simulink model "raspberrypi_audioVisualizer"  (R2018b)
settings: Solver=ode3  StartTime=0.0  StopTime=10  RelTol=1e-3  EnableMultiTasking=on
libraries: dspmtrx3 x2, sensehatlib x1, embdlinuxlib x1, raspberrypilib x1, dspxfrm3 x1
settings Model: FPTRunName=Active  ExtModeTrigDuration=2  Creator=The MathWorks, Inc.  LastModifiedBy=The MathWorks, Inc.
settings SolverCC: PositivePriorityOrder=on
settings DataIOCC: LimitDataPoints=on  SaveFormat=Array
settings OptimizationCC: ExpressionDepthLimit=2147483647  LifeSpan=Inf  MaxStackSize=64
settings DebuggingCC: UnderspecifiedInitializationDetection=Classic  MergeDetectMultiDrivingBlocksExec=none  FcnCallInpInsideContextMsg=warning  AllowSymbolicDim=off  StateNameClashWarn=warning  SFUnexpectedBacktrackingDiag=warning  SFNoUnconditionalDefaultTransitionDiag=warning  SFExecutionAtInitializationDiag=none
settings HardwareCC: ProdBitPerPointer=32  ProdBitPerSizeT=32  ProdBitPerPtrDiffT=32  ProdLargestAtomicInteger=Long  ProdLargestAtomicFloat=Double  ProdWordSize=32  ProdHWDeviceType=ARM Compatible->ARM Cortex  UseEmbeddedCoderFeatures=off  UseSimulinkCoderFeatures=off
settings ModelReferenceCC: PropagateSignalLabelsOutOfModel=off
settings SFSimCC: SimUseLocalCustomCode=off
settings RTWCC: SystemTargetFile=ert.tlc  HardwareBoard=Raspberry Pi  TemplateMakefile=ert_default_tmf  GenerateReport=on  RTWVerbose=off  RTWUseLocalCustomCode=off  Toolchain=GNU GCC Raspberry Pi  BuildConfiguration=Faster Runs  LaunchReport=on
settings CodeAppCC: ForceParamTrailComments=on  OperatorAnnotations=on  StateflowObjectComments=on  MATLABSourceComments=on
settings ERTTargetCC: MultiwordLength=2048  ERTCustomFileBanners=off  SupportContinuousTime=on  SupportNonInlinedSFcns=on  RemoveResetFunc=off  SupportVariableSizeSignals=on  ModelStepFunctionPrototypeControlCompliant=off
settings ConfigComp: CovMetricSettings=dw  CovHtmlReporting=on  CovSaveCumulativeToWorkspaceVar=on  CovSaveSingleToWorkspaceVar=on  CovExternalEMLEnable=off  CovSFcnEnable=off

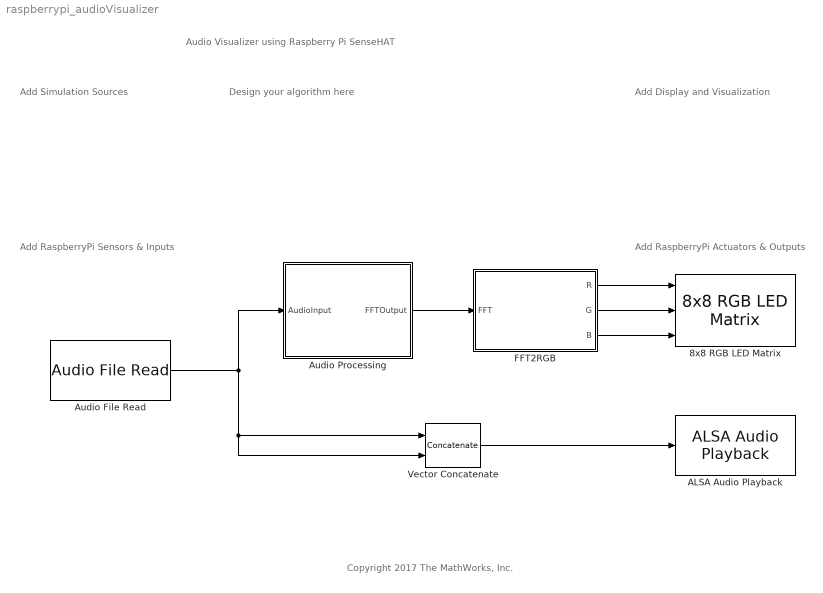
== system raspberrypi_audioVisualizer ==
  note: Copyright 2017 The MathWorks, Inc.
  note: Add Simulation Sources
  note: Add Display and Visualization
  note: Design your algorithm here
  note: Add RaspberryPi Actuators & Outputs
  note: Audio Visualizer using Raspberry Pi SenseHAT
  note: Add RaspberryPi Sensors & Inputs
  8x8 RGB LED Matrix : sensehatlib/8x8 RGB LED Matrix   Mode=Display Image  ImageSource=Separate color signals  OrientationSource=Block dialog  LEDOrientation=0  blockPlatform=Raspberry pi
      settings: SourceProductName=Simulink Support Package for Raspberry Pi Hardware  SourceProductBaseCode=RASPPI
  ALSA Audio Playback : embdlinuxlib/ALSA Audio Playback  deviceStr='hw:0,0'  sampleRateEnum=44100  queueDuration=0.5  blockPlatform=Raspberry Pi
      settings: SourceProductName=Simulink Support Package for Raspberry Pi Hardware  SourceProductBaseCode=RASPPI
  Audio File Read : raspberrypilib/Audio File Read  FileName=guitartune.wav  PlayCount=Inf  OutputEOFIndicator=off  SamplesPerFrame=8192
      settings: SourceProductName=Simulink Support Package for Raspberry Pi Hardware  SourceProductBaseCode=RASPPI
  Audio Processing : Subsystem
  FFT2RGB : MATLAB Function  TreatAsAtomicUnit=on
  Vector Concatenate : Concatenate  Mode=Multidimensional array  ConcatenateDimension=2
  wires:
  Audio File Read/1 -> Vector Concatenate/2, Vector Concatenate/1, Audio Processing/1(AudioInput)
  Vector Concatenate/1 -> ALSA Audio Playback/1
  FFT2RGB/1(R) -> 8x8 RGB LED Matrix/1
  FFT2RGB/2(G) -> 8x8 RGB LED Matrix/2
  FFT2RGB/3(B) -> 8x8 RGB LED Matrix/3
  Audio Processing/1(FFTOutput) -> FFT2RGB/1(FFT)

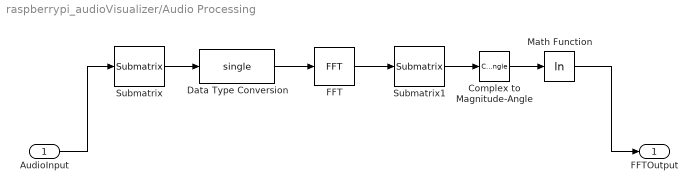
== system raspberrypi_audioVisualizer/Audio Processing ==
  AudioInput : Inport
  Complex to Magnitude-Angle : ComplexToMagnitudeAngle  Output=Magnitude
  Data Type Conversion : DataTypeConversion  OutDataTypeStr=single
  FFT : dspxfrm3/FFT  FFTImplementation=Auto  CompMethod=Table lookup  TableOpt=NEW  TableOptActive=Speed  BitRevOrder=off  Normalize=on  InheritFFTLength=on  FFTLength=64  WrapInput=on  roundingMode=Floor  overflowMode=off  firstCoeffDataTypeStr=Inherit: Same word length as input  firstCoeffLastDataTypeStr=Inherit: Same word length as input  outputMin=[]  outputMax=[]
  Math Function : Math  Operator=log  SaturateOnIntegerOverflow=on
  Submatrix : dspmtrx3/Submatrix  RowSpan=Range of rows  RowStartMode=First  RowStartIndex=1  RowEndMode=Last  RowEndIndex=1  ColSpan=One column  ColStartMode=First  ColStartIndex=1  ColEndMode=Last  ColEndIndex=1
  Submatrix1 : dspmtrx3/Submatrix  RowSpan=Range of rows  RowStartMode=Index  RowStartIndex=128  RowEndMode=Index  RowEndIndex=1151  ColSpan=Range of columns  ColStartMode=First  ColStartIndex=1  ColEndMode=Last  ColEndIndex=1
  FFTOutput : Outport
  wires:
  AudioInput/1 -> Submatrix/1
  Submatrix/1 -> Data Type Conversion/1
  Data Type Conversion/1 -> FFT/1
  FFT/1 -> Submatrix1/1
  Submatrix1/1 -> Complex to Magnitude-Angle/1
  Math Function/1 -> FFTOutput/1
  Complex to Magnitude-Angle/1 -> Math Function/1

== matlab function raspberrypi_audioVisualizer/FFT2RGB ==
  data: FFT input; R output; G output; B output
function [R,G,B] = FFT2RGB(FFT)
% Map the freqency spectrum to 8x8 led matrix in SenseHAT
% Algorithm:
% 1024 samples from frequency response is mapped to 8x8 matrix.
% Divide the fft output into 8 groups with 128 samples each.
% 
% Define maximum value for Decibels relative to full scale(dbFS)
dbFSMaxVal = 7;
% Reshape the 1024x1 fft output to 128x8 
freqMatrix = reshape(FFT,[128,8])';
% Average along the column 
avgFFT = mean(freqMatrix,2);
% Calculate LED bar length based on the average value.
% LED length = (averageFFT * 8) / Max of dbFS
ledBar = (avgFFT.*8)./dbFSMaxVal;
% Ensure ledBar will be greater than 0.
% Glithches in audio may result in negative values.
ledBar(ledBar<0) = 0;
% Atlease 1 LED should glow all time and limit the max to 8
ledBar = ledBar + 1;
ledBar(ledBar>8) = 8;
ledBar = uint8(ledBar);

% MAP the LED bar length to pixel values.
% Top(3 rows) : RED
% Middle (2 rows) : YELLOW
% Bottom (3 rows) : GREEN
% Create dummy matrix with this and get the LED matrix
LEDMatrix = zeros(8,8,'uint8');
for i = 1:8
    LEDMatrix(9-ledBar(i):8,i) = uint8(1); 
end
a = uint8([255   255   255   255   255   255   255   255;...
           255   255   255   255   255   255   255   255;...
           255   255   255   255   255   255   255   255;...
           128   128   128   128   128   128   128   128;...
           128   128   128   128   128   128   128   128;...
           0     0     0     0     0     0     0     0;...
           0     0     0     0     0     0     0     0;...
           0     0     0     0     0     0     0     0;...
           ]);
       
b = uint8([0     0     0     0     0     0     0     0;...
           0     0     0     0     0     0     0     0;...
           0     0     0     0     0     0     0     0;...
           128   128   128   128   128   128   128   128;...
           128   128   128   128   128   128   128   128;...
           255   255   255   255   255   255   255   255;...
           255   255   255   255   255   255   255   255;...
           255   255   255   255   255   255   255   255;...
           ]);
       
c = zeros(8,8,'uint8');

R = a.*LEDMatrix;
G = b.*LEDMatrix;
B = c;
